simulink model "Program1"  (Simulink 9.0)
settings: Solver=FixedStepDiscrete  StartTime=0.0  StopTime=10.0  RelTol=1e-3  EnableMultiTasking=on
values from neighbouring files (symbols this model uses):
  K_PWM = 8.087    [ModelDD.m]
  l = 0.12    [ModelDD.m]
  R = 0.027    [ModelDD.m]
undefined symbols (not defined in the file or in its folder): DiscIntNeverNeededParam
libraries: legoev3lib x4, simulink x3
settings Model: Creator=ACER  LastModifiedBy=USER  ExtModeTrigDuration=2
settings SolverCC: PositivePriorityOrder=on  AutoInsertRateTranBlk=on
settings DataIOCC: SaveFormat=Dataset  ReturnWorkspaceOutputs=on
settings OptimizationCC: UseDivisionForNetSlopeComputation=on  UseFloatMulNetSlope=on  PassReuseOutputArgsAs=Individual arguments  ZeroExternalMemoryAtStartup=off  ZeroInternalMemoryAtStartup=off  NoFixptDivByZeroProtection=on  EfficientFloat2IntCast=on  LifeSpan=1  MaxStackSize=64
settings DebuggingCC: AlgebraicLoopMsg=none  UnderspecifiedInitializationDetection=Simplified  MergeDetectMultiDrivingBlocksExec=error  ParameterTunabilityLossMsg=error  SFUnexpectedBacktrackingDiag=error  SFNoUnconditionalDefaultTransitionDiag=error  SFExecutionAtInitializationDiag=warning
settings HardwareCC: ProdLargestAtomicInteger=Long  ProdLargestAtomicFloat=Float  ProdIntDivRoundTo=Zero  ProdEndianess=LittleEndian  ProdHWDeviceType=ARM Compatible->ARM 9
settings ModelReferenceCC: PropagateSignalLabelsOutOfModel=on
settings SFSimCC: SimUseLocalCustomCode=on  MATLABDynamicMemAlloc=off
settings RTWCC: SystemTargetFile=ert.tlc  HardwareBoard=LEGO MINDSTORMS EV3  TLCOptions="-aInlineSetEventsForThisBaseRateFcn=TLC_FALSE -aSuppressMultiTaskScheduler=TLC_FALSE  -aRateBasedStepFcn=0"  TemplateMakefile=ert_default_tmf  Description=Embedded Coder  GenerateReport=on  RTWUseLocalCustomCode=on  Toolchain=Sourcery G++ Lite v2009q3  IncludeHyperlinkInReport=on  LaunchReport=on  GenerateTraceInfo=on  GenerateTraceReport=on  GenerateTraceReportSl=on  GenerateTraceReportSf=on  GenerateTraceReportEml=on  GenerateCodeMetricsReport=on
settings MATStruct: className=codertarget.tools.BuildHook  argsTopModelOnly=[]  excludedModels=[]  includeReferencedModels=on  includeTopModel=on  enabled=on  UseCoderTarget=[1]  TargetHardware=LEGO MINDSTORMS EV3  RTOS=Linux  RTOSBaseRateTaskPriority=40  DetectTaskOverruns=[0.0]  Scheduler_interrupt_source=[0.0]  DataVersion=2016.02  IPAddress=codertarget.ev3.internal.getEV3ExtmodeIPaddr  Port=17725  Verbose=[0]  Configuration=TCP/IP  Running=[0.0]  BuildAction=Build, load and run  type=USB  deviceID=0016534b0c89  IPAddressCpy=192.168.43.195
settings CodeAppCC: ForceParamTrailComments=on  IgnoreCustomStorageClasses=off  OperatorAnnotations=on  SimulinkDataObjDesc=on  SFDataObjDesc=on  CustomSymbolStrGlobalVar=rt$N$M  CustomSymbolStrType=$N$M  CustomSymbolStrFcn=$N$M$F  CustomSymbolStrMacro=$N$M  InsertBlockDesc=on  StateflowObjectComments=off
settings ERTTargetCC: IncludeMdlTerminateFcn=off  CombineSignalStateStructs=on  SupportAbsoluteTime=off  SupportComplex=off  SupportContinuousTime=on  SupportNonInlinedSFcns=on  SupportVariableSizeSignals=on  ERTFilePackagingFormat=CompactWithDataFile
settings ConfigComp: CovMetricSettings=dwe  CovHtmlReporting=off  CovSaveCumulativeToWorkspaceVar=off  CovSaveSingleToWorkspaceVar=off  CovExternalEMLEnable=on

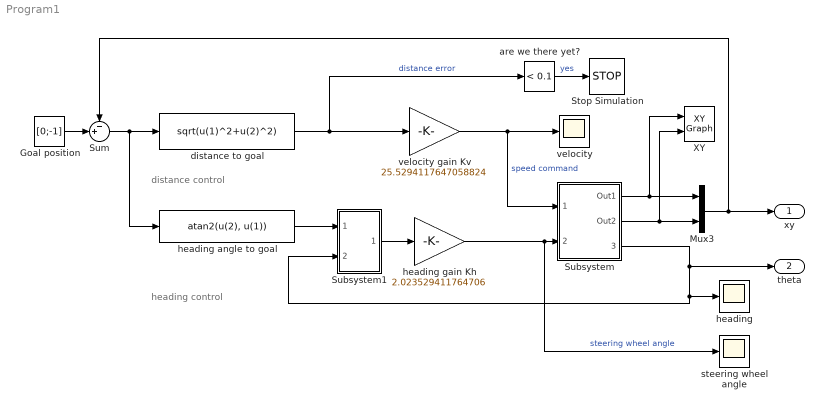
== system Program1 ==
  note: distance control
  note: heading control
  Goal position : Constant  Value=[0;-1]
  Mux3 : Mux  Inputs=2
  Stop Simulation : Stop
  Subsystem : Subsystem
  Subsystem1 : Subsystem
  Sum : Sum  Inputs=-+|
  XY : simulink/Sinks/XY Graph  xmin=-6  xmax=6  ymin=-6  ymax=6  st=-1
  are we there yet? : simulink/Logic and Bit Operations/Compare To Constant  relop=<  const=0.1  OutDataTypeStr=boolean
  distance to goal : Fcn  Expr=sqrt(u(1)^2+u(2)^2)
  heading : Scope
  heading angle to goal : Fcn  Expr=atan2(u(2), u(1))
  heading gain Kh : Gain  Gain=2.023529411764706
  steering wheel angle : Scope
  velocity : Scope
  velocity gain Kv : Gain  Gain=25.5294117647058824
  xy : Outport
  "theta " : Outport  Port=2
  wires:
  Goal position/1 -> Sum/2
  are we there yet?/1 -> Stop Simulation/1  "yes"
  Mux3/1 -> xy/1, Sum/1
  distance to goal/1 -> velocity gain Kv/1, are we there yet?/1  "distance error"
  heading gain Kh/1 -> Subsystem/2(steering wheel angle), steering wheel angle/1  "steering wheel angle"
  velocity gain Kv/1 -> Subsystem/1(speed command), velocity/1  "speed command"
  Sum/1 -> distance to goal/1, heading angle to goal/1
  Subsystem/2(Out2) -> Mux3/2, XY/2
  Subsystem/1(Out1) -> Mux3/1, XY/1
  Subsystem/3(current heading) -> Subsystem1/2(In2), heading/1, "theta "/1
  heading angle to goal/1 -> Subsystem1/1(In1)
  Subsystem1/1(heading error) -> heading gain Kh/1

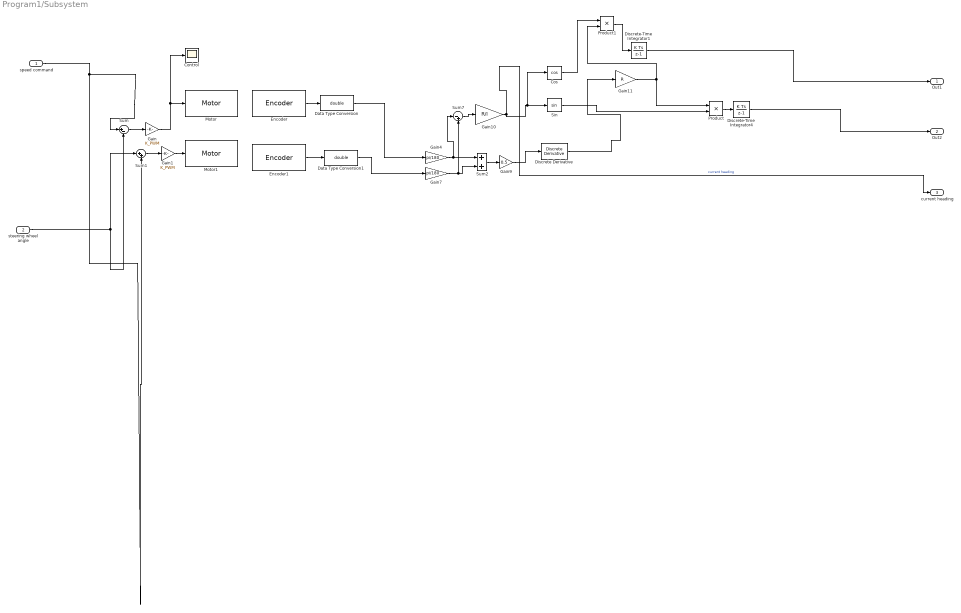
== system Program1/Subsystem ==
  speed command : Inport
  steering wheel angle : Inport  Port=2
  Control : Scope
  Cos : Trigonometry  Operator=cos
  Data Type Conversion : DataTypeConversion  OutDataTypeStr=double
  Data Type Conversion1 : DataTypeConversion  OutDataTypeStr=double
  Discrete Derivative : simulink/Discrete/Discrete Derivative  gainval=1.0  ICPrevScaledInput=0.0  OutMin=[]  OutMax=[]  OutDataType=fixdt(1, 16)  OutScaling=2^-10  DoSatur=off
  Discrete-Time Integrator1 : DiscreteIntegrator  InitialConditionSetting=State (most efficient)  SampleTime=0.033  ICPrevOutput=DiscIntNeverNeededParam  ICPrevScaledInput=DiscIntNeverNeededParam
  Discrete-Time Integrator4 : DiscreteIntegrator  InitialConditionSetting=State (most efficient)  SampleTime=0.033  ICPrevOutput=DiscIntNeverNeededParam  ICPrevScaledInput=DiscIntNeverNeededParam
  Encoder : legoev3lib/Encoder  portNumber=B  opMode=No reset  sampleTime=Ts
      settings: SourceProductName=Simulink Support Package for LEGO MINDSTORMS EV3 Hardware  SourceProductBaseCode=LEGOEV3
  Encoder1 : legoev3lib/Encoder  portNumber=C  opMode=No reset  sampleTime=Ts
      settings: SourceProductName=Simulink Support Package for LEGO MINDSTORMS EV3 Hardware  SourceProductBaseCode=LEGOEV3
  Gain : Gain  Gain=K_PWM
  Gain1 : Gain  Gain=K_PWM
  Gain10 : Gain  Gain=R/l
  Gain11 : Gain  Gain=R
  Gain4 : Gain  Gain=pi/180
  Gain7 : Gain  Gain=pi/180
  Gain9 : Gain  Gain=0.5
  Motor : legoev3lib/Motor  sportNumber=B  sstopAction=Brake
  Motor1 : legoev3lib/Motor  sportNumber=C  sstopAction=Brake
  Product : Product
  Product1 : Product
  Sin : Trigonometry
  Sum : Sum  Inputs=|+-
  Sum1 : Sum  Inputs=|++
  Sum2 : Sum
  Sum7 : Sum  Inputs=|-+
  Out1 : Outport
  Out2 : Outport  Port=2
  current heading : Outport  Port=3
  wires:
  steering wheel angle/1 -> Sum1/1, Sum/2
  speed command/1 -> Sum1/2, Sum/1
  Discrete-Time Integrator1/1 -> Out1/1
  Gain10/1 -> Cos/1, Sin/1, current heading/1  "current heading"
  Sum7/1 -> Gain10/1
  Gain11/1 -> Product/1, Product1/2
  Product1/1 -> Discrete-Time Integrator1/1
  Gain7/1 -> Sum7/2, Sum2/2
  Discrete Derivative/1 -> Gain11/1
  Gain9/1 -> Discrete Derivative/1
  Product/1 -> Discrete-Time Integrator4/1
  Gain4/1 -> Sum7/1, Sum2/1
  Sin/1 -> Product/2
  Discrete-Time Integrator4/1 -> Out2/1
  Cos/1 -> Product1/1
  Sum2/1 -> Gain9/1
  Sum1/1 -> Gain1/1
  Encoder/1 -> Data Type Conversion/1
  Encoder1/1 -> Data Type Conversion1/1
  Sum/1 -> Gain/1
  Data Type Conversion/1 -> Gain4/1
  Data Type Conversion1/1 -> Gain7/1
  Gain/1 -> Motor/1, Control/1
  Gain1/1 -> Motor1/1

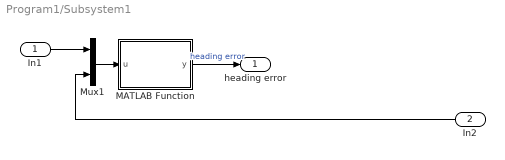
== system Program1/Subsystem1 ==
  In1 : Inport
  In2 : Inport  Port=2
  MATLAB Function : MATLAB Function  TreatAsAtomicUnit=on
  Mux1 : Mux  Inputs=2
  heading error : Outport
  wires:
  In2/1 -> Mux1/2
  In1/1 -> Mux1/1
  MATLAB Function/1(y) -> heading error/1  "heading error"
  Mux1/1 -> MATLAB Function/1(u)

== matlab function Subsystem1/MATLAB Function ==
  data: u input double; y output double
function y = fcn(u)

y = angdiff(u(2),u(1));
